simulink model "EX2_Pend_up_Controller_Observer"  (R2023b)
settings: Solver=FixedStepDiscrete  StartTime=0.0  StopTime=Inf  FixedStep=Ts  RelTol=1e-3  EnableMultiTasking=on
model workspace (MATLAB code in the model file):
  | % Processor Frequency
  | CPU_frequency = 90e6; %(Hz)
  | 
  | % PWM Settings
  | PWM_frequency = 15e3; %(Hz)
  | PWM_CounterPeriod = CPU_frequency/PWM_frequency/2; %(PWM timer counts)
  | 
  | % Switching frequency
  | fsw = PWM_frequency;
  | 
  | % Integration time (solver)
  | Ts = 1e-4;
  | 
  | % Encoder settings
  | fw = 400; % encoder sampling frequency
  | Tw = 1/fw; % encoder sampling time
values from neighbouring files (symbols this model uses):
  A = [0, 1, 0, 0 ... (first row only)    [EX2_init.m]
  Ad = sys_obs_disc.A    [EX2_init.m]
  B = Kf_avg * B    [EX2_init.m]
  Bd = sys_obs_disc.B    [EX2_init.m]
  C = [1, 0, 0, 0 ... (first row only)    [EX2_init.m]
  c_gains = K    [EX2_init.m]
  CALIBRATION_TIME = 50    [EX2_init.m]
  Cd = sys_obs_disc.C    [EX2_init.m]
  Dd = sys_obs_disc.D    [EX2_init.m]
  K = place(A, B, P_K)    [EX2_init.m]
  K_e = Distance / Encoder_Counts    (= 0.000124665903016)    [EX2_init.m]
  Lc = place(A', C', P_L)'    [EX2_init.m]
  SMC_switch = 1    [EX2_init.m]
  sys_params = [params.M, params.m, params.L, params.I, params.b_dynamic, params.bp_dynamic, params.g, K_sw]    [EX2_init.m]
undefined symbols (not defined in the file or in its folder): DiscIntNeverNeededParam, Down, GPTRIP1SEL, GPTRIP2SEL, TZ1, TZ2, Up
libraries: c2802xlib x5, eeGeneralControl x2, c2806xlib x2, dspstat3 x2, c280xlib x1, simulink x1, dspfdesign x1, dspsigops x1
settings Model: ExtModeTrigDuration=8  Creator=The MathWorks, Inc.  LastModifiedBy=98912
settings SolverCC: AlgebraicLoopSolver=TrustRegion  AutoInsertRateTranBlk=on
settings OptimizationCC: DefaultUnderspecifiedDataType=single  EnhancedBackFolding=on  PassReuseOutputArgsAs=Individual arguments  MaxStackSize=1024  OptimizeBlockOrder=speed  DifferentSizesBufferReuse=on  OptimizationCustomize=off  DenormalBehavior=FlushToZero  EfficientTunableParamExpr=on
settings DebuggingCC: ParameterTunabilityLossMsg=error  UnconnectedInputMsg=warning  UnconnectedOutputMsg=warning  UnconnectedLineMsg=warning  SubsystemReferenceDiagnosticForUnitTest=warning
settings HardwareCC: ProdBitPerChar=16  ProdBitPerInt=16  ProdBitPerPointer=32  ProdBitPerSizeT=32  ProdBitPerPtrDiffT=32  ProdLargestAtomicInteger=Integer  ProdLargestAtomicFloat=None  ProdWordSize=16  ProdLongLongMode=on  ProdHWDeviceType=Texas Instruments->C2000
settings ModelReferenceCC: EnableRefExpFcnMdlSchedulingChecks=on
settings SFSimCC: MATLABDynamicMemAlloc=off
settings RTWCC: Description=Embedded Coder  SystemTargetFile=ert.tlc  HardwareBoard=TI Piccolo F28069M LaunchPad  TemplateMakefile=ert_default_tmf  GenerateReport=on  Toolchain=Texas Instruments Code Composer Studio (C2000)  DLArmComputeVersion=19.05
settings CodeAppCC: ForceParamTrailComments=on  IgnoreCustomStorageClasses=off  OperatorAnnotations=on  SimulinkDataObjDesc=on  SFDataObjDesc=on  InsertBlockDesc=on
settings ERTTargetCC: CodeReplacementLibrary=TI C28x  ExtModeStaticAllocSize=2000
settings SettingsController: UseSoCProfilerForTargets=0

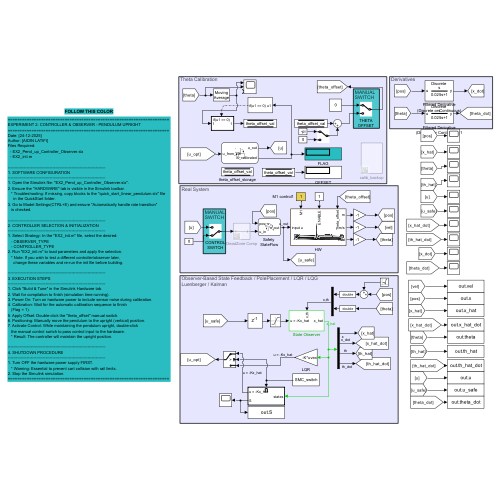
[thumbnail: Simulink's stored preview of the top-level diagram]
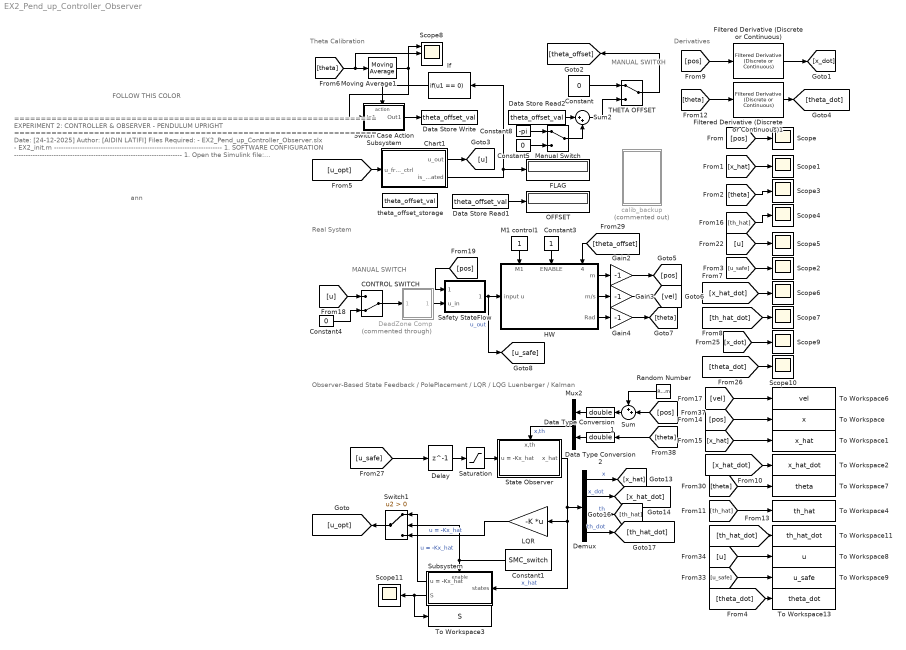
== system EX2_Pend_up_Controller_Observer ==
  note: FOLLOW THIS COLOR
  note: MANUAL
      | SWITCH
  note: MANUAL
      | SWITCH
  note: ====================================================================
      | EXPERIMENT 2: CONTROLLER & OBSERVER - PENDULUM UPRIGHT
      | ====================================================================
      | Date: [24-12-2025]
      | Author: [AIDIN LATIFI]
      | Files Required:
      |   - EX2_Pend_up_Controller_Observer.slx
      |   - EX2_init.m
      |
      | ------------------------------------------------------------------------
      | 1. SOFTWARE CONFIGURATION
      | ------------------------------------------------------------------------
      | 1. Open the Simulink file: "EX2_Pend_up_Controller_Observer.slx".
      | 2. Ensure the "HARDWARE" tab is visible in the Simulink toolbar.
      |    * Troubleshooting: If missing, copy blocks to the "quick_start_linear_pendulum.slx" file
      |      in the QuickStart folder.
      | 3. Go to Model Settings(CTRL+E) and ensure "Automatically handle rate transition"
      |    is checked.
      |
      | ------------------------------------------------------------------------
      | 2. CONTROLLER SELECTION & INITIALIZATION
      | ------------------------------------------------------------------------
      | 1. Select Strategy: In the "EX2_init.m" file, select the desired:
      |    - OBSERVER_TYPE
      |    - CONTROLLER_TYPE
      | 2. Run "EX2_init.m" to load parameters and apply the selection.
      |    * Note: If you wish to test a different controller/observer later,
      |      change these variables and re-run the init file before building.
      |
      | ------------------------------------------------------------------------
      | 3. EXECUTION STEPS
      | ------------------------------------------------------------------------
      | 1. Click "Build & Tune" in the Simulink Hardware tab.
      | 2. Wait for compilation to finish (simulation time running).
      | 3. Power On: Turn on hardware power to include sensor noise during calibration.
      | 4. Calibration: Wait for the automatic calibration sequence to finish
      |    (Flag = 1).
      | 5. Apply Offset: Double-click the "theta_offset" manual switch.
      | 6. Positioning: Manually move the pendulum to the upright (vertical) position.
      | 7. Activate Control: While maintaining the pendulum upright, double-click
      |    the manual control switch to pass control input to the hardware.
      |    * Result: The controller will maintain the upright position.
      |
      | ------------------------------------------------------------------------
      | 4. SHUTDOWN PROCEDURE
      | ------------------------------------------------------------------------
      | 1. Turn OFF the hardware power supply FIRST.
      |    * Warning: Essential to prevent cart collision with rail limits.
      | 2. Stop the Simulink simulation.
      | ====================================================================
  note: ann
  note: Theta Calibration
  note: Observer-Based State Feedback / PolePlacement / LQR / LQG
      | Luenberger / Kalman
  note: Real System
  note: Derivatives
  CONTROL SWITCH : ManualSwitch  CurrentSetting=0
  Chart1 : Stateflow chart  TreatAsAtomicUnit=on
  Constant : Constant  Value=0  SampleTime=Ts
  Constant1 : Constant  Value=SMC_switch
  Constant3 : Constant
  Constant4 : Constant  Value=0  SampleTime=-1
  Constant5 : Constant  Value=0  SampleTime=Ts
  Constant8 : Constant  Value=-pi  SampleTime=Ts
  Data Store Read1 : DataStoreRead  DataStoreName=theta_offset_val  IndexOptions=Index vector (dialog)  Indices=1  OutputSizes=1
  Data Store Read2 : DataStoreRead  DataStoreName=theta_offset_val  IndexOptions=Index vector (dialog)  Indices=1  OutputSizes=1
  Data Store Write : DataStoreWrite  DataStoreName=theta_offset_val  IndexOptions=Index vector (dialog)  Indices=1  OutputSizes=1
  Data Type Conversion1 : DataTypeConversion  OutDataTypeStr=double  SaturateOnIntegerOverflow=off  RndMeth=Floor
  Data Type Conversion2 : DataTypeConversion  OutDataTypeStr=double  SaturateOnIntegerOverflow=off  RndMeth=Floor
  DeadZone Comp : Subsystem  Commented=through
  Delay : Delay  DelayLength=1  SampleTime=Ts
  Demux : Demux
  FLAG : Display
  Filtered Derivative (Discrete or Continuous) : eeGeneralControl/Filtered Derivative (Discrete or Continuous)  K=1  T=0.025  B=inf  A=-inf  minRatio=10  init_option=Inherited from block input  x0=0  Ts=-1
      settings: LibrarySourceBlock=|
      | ee_sl_lib/General Control/Filtered Derivative
      | (Discrete or Continuous)
  Filtered Derivative (Discrete or Continuous)1 : eeGeneralControl/Filtered Derivative (Discrete or Continuous)  K=1  T=0.025  B=inf  A=-inf  minRatio=10  init_option=Inherited from block input  x0=0  Ts=-1
      settings: LibrarySourceBlock=|
      | ee_sl_lib/General Control/Filtered Derivative
      | (Discrete or Continuous)
  Gain2 : Gain  Gain=-1
  Gain3 : Gain  Gain=-1
  Gain4 : Gain  Gain=-1
  HW : Subsystem
      settings: PortSchema="{\"entries\":[{\"content\":{\"sides\":[{\"content\":{\"connectorIds\":[\"In1\"]},\"type\":\"ConnectorPlacement.EquallySpacedRectSide\",\"uuid\":\"e9898c75-a6e7-4646-b73a-b35b1fbe5adf\"},{\"content\":{\"connectorIds\":[\"Out1\",\"Out2\",\"Out3\"],\"side\":\"RIGHT\"},\"type\":\"ConnectorPlacement.EquallySpacedRectSide\",\"uuid\":\"085d2ccc-0e1f-4b16-8ec9-c70e62f660a1\"},{\"content\":{\"connectorIds\":[\"In2\",\"In3\",\"In4\"],\"side\":\"TOP\"},\"type\":\"ConnectorPlacement.EquallySpacedRectSide\",\"uuid\":\"51882789-74c2-4a7a-a001-ddaf25b9b479\"}]},\"type\":\"ConnectorPlacement.EquallySpacedConnector\",\"uuid\":\"373898fa-4a42-48b4-8ce1-77edd11dc4d5\"}],\"packageUris\":[\"http://schema.mathworks.com/mf0/Connector/R2020b\"],\"version\":\"1.0\"}"
      mask Display: image('lineer_pendulum_v2.jpg');
  If : If  IfExpression=u1 == 0  ShowElse=off
  LQR : Gain  Gain=-K  Multiplication=Matrix(K*u) (u vector)
  M1 control1 : Constant
  Manual Switch : ManualSwitch
  Moving Average1 : dspstat3/Moving Average  Method=Sliding window  ForgettingFactorPort=off  SpecifyWindowLength=off  WindowLength=200  OverlapLength=5  AllowArbitraryInputLength=off  ForgettingFactor=0.9  SimulateUsing=Interpreted execution
  Mux2 : Mux  Inputs=2
  OFFSET : Display
  Random Number : RandomNumber  Variance=1e-9
  Safety StateFlow : Stateflow chart  TreatAsAtomicUnit=on
  Saturation : Saturate  UpperLimit=1  LowerLimit=-1
  Scope{,1..7,9..11} (11 alike) : Scope
  Scope8 : Scope  NumInputPorts=3
  State Observer : Subsystem
      settings: PortSchema="{\"entries\":[{\"content\":{\"sides\":[{\"content\":{\"connectorIds\":[\"In1\"]},\"type\":\"ConnectorPlacement.EquallySpacedRectSide\",\"uuid\":\"78a5d6cc-05c3-4998-83bd-765592313900\"},{\"content\":{\"connectorIds\":[\"Out1\"],\"side\":\"RIGHT\"},\"type\":\"ConnectorPlacement.EquallySpacedRectSide\",\"uuid\":\"01493a4c-d438-46a2-bc76-28dd63b6a3eb\"},{\"content\":{\"connectorIds\":[\"In2\"],\"side\":\"TOP\"},\"type\":\"ConnectorPlacement.EquallySpacedRectSide\",\"uuid\":\"8eaa5f99-6d7d-4ceb-8f85-a6d0adbc0832\"}]},\"type\":\"ConnectorPlacement.EquallySpacedConnector\",\"uuid\":\"d4438f88-f341-4cd2-b661-553fe6a2df92\"}],\"packageUris\":[\"http://schema.mathworks.com/mf0/Connector/R2020b\"],\"version\":\"1.0\"}"
  Subsystem : Subsystem
  Sum : Sum  Inputs=++|
  Sum2 : Sum  Inputs=|++
  Switch Case Action Subsystem : Subsystem  TreatAsAtomicUnit=on
  Switch1 : Switch  Criteria=u2 > Threshold  SaturateOnIntegerOverflow=off  InputSameDT=off
  THETA OFFSET : ManualSwitch
  To Workspace : ToWorkspace  VariableName=x  SaveFormat=Timeseries  SampleTime=-1
  To Workspace1 : ToWorkspace  VariableName=x_hat  SaveFormat=Timeseries  SampleTime=-1
  To Workspace11 : ToWorkspace  VariableName=th_hat_dot  SaveFormat=Timeseries  SampleTime=-1
  To Workspace13 : ToWorkspace  VariableName=theta_dot  SaveFormat=Timeseries  SampleTime=-1
  To Workspace2 : ToWorkspace  VariableName=x_hat_dot  SaveFormat=Timeseries  SampleTime=-1
  To Workspace3 : ToWorkspace  VariableName=S  SaveFormat=Timeseries  SampleTime=-1
  To Workspace4 : ToWorkspace  VariableName=th_hat  SaveFormat=Timeseries  SampleTime=-1
  To Workspace6 : ToWorkspace  VariableName=vel  SaveFormat=Timeseries  SampleTime=-1
  To Workspace7 : ToWorkspace  VariableName=theta  SaveFormat=Timeseries  SampleTime=-1
  To Workspace8 : ToWorkspace  VariableName=u  SaveFormat=Timeseries  SampleTime=-1
  To Workspace9 : ToWorkspace  VariableName=u_safe  SaveFormat=Timeseries  SampleTime=-1
  calib_backup : Subsystem  Commented=on
  theta_offset_storage : DataStoreMemory  DataStoreName=theta_offset_val  WriteAfterWriteMsg=warning  ShowAdditionalParam=off
  wires:
  [u_safe] -> Scope2/1
  Constant8/1 -> Manual Switch/1
  If/1 -> Switch Case Action Subsystem/Action
  [u_opt] -> Chart1/1(u_from_ctrl)
  [theta] -> Filtered Derivative (Discrete or Continuous)1/1
  Constant/1 -> THETA OFFSET/1
  Constant4/1 -> CONTROL SWITCH/2
  THETA OFFSET/1 -> [theta_offset]
  Sum2/1 -> THETA OFFSET/2
  [th_hat_dot] -> To Workspace11/1
  [theta] -> Scope8/2, Moving Average1/1
  [theta] -> Data Type Conversion2/1
  Switch Case Action Subsystem/1(Out1) -> Data Store Write/1
  [x_hat_dot] -> To Workspace2/1
  Manual Switch/1 -> Sum2/2
  Safety StateFlow/1(u_out) -> HW/1(input u), [u_safe]  "u_out"
  HW/3(Rad) -> Gain4/1
  Chart1/2(is_calibrated) -> FLAG/1, If/1
  [th_hat] -> To Workspace4/1
  Sum/1 -> Data Type Conversion1/1
  [pos] -> To Workspace/1
  Constant3/1 -> HW/3(ENABLE)
  M1 control1/1 -> HW/2(M1)
  Random Number/1 -> Sum/1
  Demux/1 -> [x_hat]  "x"
  [u] -> Scope5/1
  [x_hat] -> To Workspace1/1
  Demux/2 -> [x_hat_dot]  "x_dot"
  CONTROL SWITCH/1 -> DeadZone Comp/1(In1)
  [pos] -> Scope/1
  HW/2(m/s) -> Gain3/1
  [pos] -> Sum/2
  LQR/1 -> Switch1/3  "u = -Kx_hat"
  Gain3/1 -> [vel]
  Chart1/1(u_out) -> [u]
  Filtered Derivative (Discrete or Continuous)/1 -> [x_dot]
  Gain2/1 -> [pos]
  [th_hat_dot] -> Scope7/1
  Constant5/1 -> Manual Switch/2
  [pos] -> Filtered Derivative (Discrete or Continuous)/1
  [theta_offset] -> HW/4(Theta_offset)
  Moving Average1/1 -> Switch Case Action Subsystem/1(In1), Scope8/1
  Filtered Derivative (Discrete or Continuous)1/1 -> [theta_dot]
  Gain4/1 -> [theta]
  Data Store Read1/1 -> OFFSET/1
  [u_safe] -> To Workspace9/1
  [theta] -> Scope3/1
  [x_hat_dot] -> Scope6/1
  [pos] -> Safety StateFlow/1(pos_s)
  [x_hat] -> Scope1/1
  State Observer/1(x_hat) -> LQR/1, Subsystem/1(states), Demux/1  "x_hat"
  Demux/4 -> [th_hat_dot]  "th_dot"
  [th_hat] -> Scope4/1
  Data Type Conversion2/1 -> Mux2/2
  Mux2/1 -> State Observer/2(x,th)  "x,th"
  [vel] -> To Workspace6/1
  HW/1(m) -> Gain2/1
  [u] -> CONTROL SWITCH/1
  DeadZone Comp/1(Out1) -> Safety StateFlow/2(u_in)
  [x_dot] -> Scope9/1
  Data Type Conversion1/1 -> Mux2/1
  [theta_dot] -> To Workspace13/1
  [theta_dot] -> Scope10/1
  [theta] -> To Workspace7/1
  Demux/3 -> [th_hat]  "th"
  [u] -> To Workspace8/1
  Data Store Read2/1 -> Sum2/1
  Delay/1 -> Saturation/1
  [u_safe] -> Delay/1
  Saturation/1 -> State Observer/1(u = -Kx_hat)
  Constant1/1 -> Subsystem/Enable, Switch1/2
  Subsystem/2(S) -> To Workspace3/1, Scope11/1
  Subsystem/1(u = -Kx_hat) -> Switch1/1  "u = -Kx_hat"
  Switch1/1 -> [u_opt]

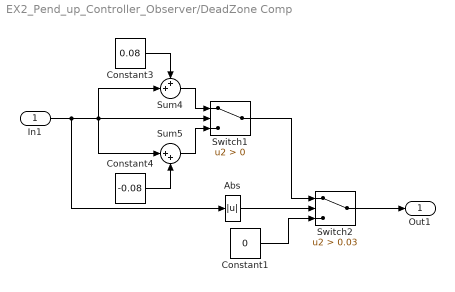
== system EX2_Pend_up_Controller_Observer/DeadZone Comp ==
  In1 : Inport
  Abs : Abs  SaturateOnIntegerOverflow=off
  Constant1 : Constant  Value=0  SampleTime=Ts
  Constant3 : Constant  Value=0.08  SampleTime=Ts
  Constant4 : Constant  Value=-0.08  SampleTime=Ts
  Sum4 : Sum  Inputs=++|
  Sum5 : Sum  Inputs=|++
  Switch1 : Switch  Criteria=u2 > Threshold  ZeroCross=off  SaturateOnIntegerOverflow=off  InputSameDT=off
  Switch2 : Switch  Criteria=u2 > Threshold  Threshold=0.03  ZeroCross=off  SaturateOnIntegerOverflow=off  InputSameDT=off
  Out1 : Outport
  wires:
  Switch2/1 -> Out1/1
  Constant1/1 -> Switch2/3
  Abs/1 -> Switch2/2
  In1/1 -> Abs/1, Switch1/2, Sum4/2, Sum5/1
  Constant4/1 -> Sum5/2
  Sum4/1 -> Switch1/1
  Switch1/1 -> Switch2/1
  Sum5/1 -> Switch1/3
  Constant3/1 -> Sum4/1

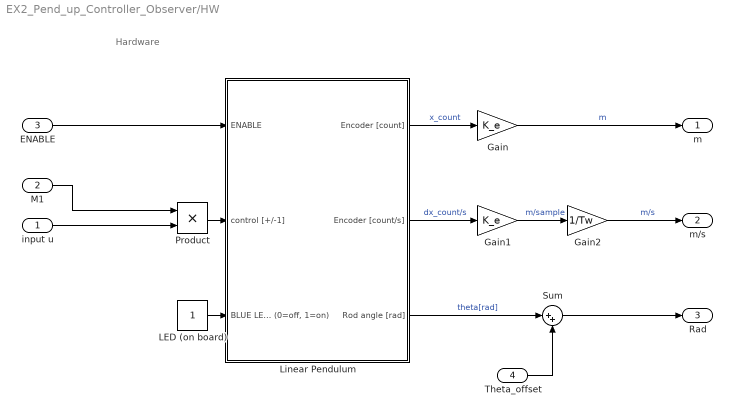
== system EX2_Pend_up_Controller_Observer/HW ==
  note: Hardware
  input u : Inport
  M1 : Inport  Port=2
  ENABLE : Inport  Port=3
  Theta_offset : Inport  Port=4
  Gain : Gain  Gain=K_e
  Gain1 : Gain  Gain=K_e
  Gain2 : Gain  Gain=1/Tw
  LED (on board) : Constant  SampleTime=0.5
  Linear Pendulum : Subsystem
  Product : Product
  Sum : Sum  Inputs=|++
  m : Outport
  m/s : Outport  Port=2
  Rad : Outport  Port=3
  wires:
  Sum/1 -> Rad/1
  Gain1/1 -> Gain2/1  "m/sample"
  Theta_offset/1 -> Sum/2
  Gain/1 -> m/1  "m"
  Gain2/1 -> m/s/1  "m/s"
  M1/1 -> Product/1
  Linear Pendulum/2(Encoder [count/s]) -> Gain1/1  "dx_count/s"
  input u/1 -> Product/2
  Linear Pendulum/3(Rod angle [rad]) -> Sum/1  "theta[rad]"
  Product/1 -> Linear Pendulum/2(control [+/-1])
  LED (on board)/1 -> Linear Pendulum/3("BLUE LED (0=off, 1=on)")
  Linear Pendulum/1(Encoder [count]) -> Gain/1  "x_count"
  ENABLE/1 -> Linear Pendulum/1(ENABLE)

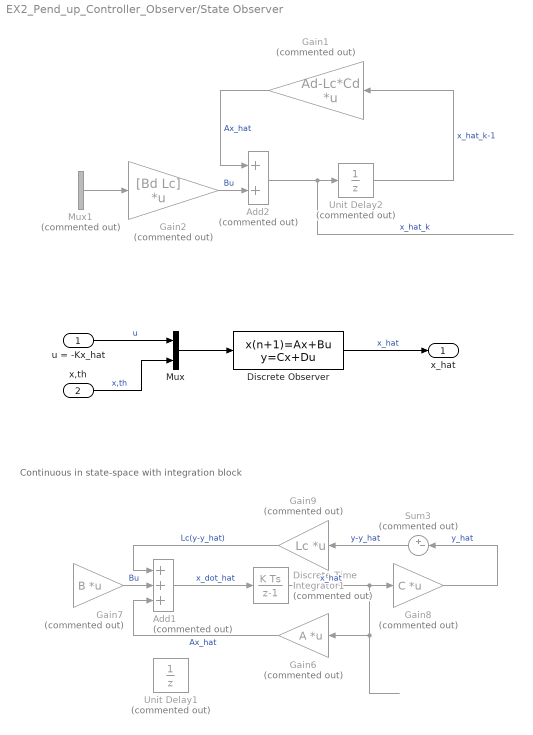
== system EX2_Pend_up_Controller_Observer/State Observer ==
  note: Continuous in state-space with integration block
  u = -Kx_hat : Inport
  x,th : Inport  Port=2
  Add1 : Sum  Commented=on  Inputs=+++
  Add2 : Sum  Commented=on
  Discrete Observer : DiscreteStateSpace  A=Ad  B=Bd  C=Cd  D=Dd  InitialCondition=[0;0;0;0]  SampleTime=Ts
  Discrete-Time Integrator1 : DiscreteIntegrator  Commented=on  InitialCondition=[0,0,0,0]  SampleTime=-1  LimitOutput=on  UpperSaturationLimit=0.01  LowerSaturationLimit=-0.01  ICPrevOutput=DiscIntNeverNeededParam  ICPrevScaledInput=DiscIntNeverNeededParam
  Gain1 : Gain  Commented=on  Gain=Ad-Lc*Cd  Multiplication=Matrix(K*u) (u vector)
  Gain2 : Gain  Commented=on  Gain=[Bd Lc]  Multiplication=Matrix(K*u) (u vector)
  Gain6 : Gain  Commented=on  Gain=A  Multiplication=Matrix(K*u) (u vector)
  Gain7 : Gain  Commented=on  Gain=B  Multiplication=Matrix(K*u) (u vector)
  Gain8 : Gain  Commented=on  Gain=C  Multiplication=Matrix(K*u) (u vector)
  Gain9 : Gain  Commented=on  Gain=Lc  Multiplication=Matrix(K*u) (u vector)
  Mux : Mux  Inputs=2
  Mux1 : Mux  Commented=on  Inputs=2
  Sum3 : Sum  Commented=on  Inputs=+-|
  Unit Delay1 : UnitDelay  Commented=on  SampleTime=-1  HasFrameUpgradeWarning=on
  Unit Delay2 : UnitDelay  Commented=on  SampleTime=-1  HasFrameUpgradeWarning=on
  x_hat : Outport
  wires:
  Gain6/1 -> Add1/3  "Ax_hat"
  Sum3/1 -> Gain9/1  "y-y_hat"
  Gain8/1 -> Sum3/2  "y_hat"
  Gain9/1 -> Add1/1  "Lc(y-y_hat)"
  Gain7/1 -> Add1/2  "Bu"
  Add1/1 -> Discrete-Time Integrator1/1  "x_dot_hat"
  Discrete-Time Integrator1/1 -> Gain6/1, Gain8/1  "x_hat"
  Mux/1 -> Discrete Observer/1
  Discrete Observer/1 -> x_hat/1  "x_hat"
  x,th/1 -> Mux/2  "x,th"
  u = -Kx_hat/1 -> Mux/1  "u"
  ? -> Sum3/1  "x,th"
  ? -> Gain7/1  "u"
  Add2/1 -> Unit Delay2/1  "x_hat_k"
  Gain2/1 -> Add2/2  "Bu"
  Gain1/1 -> Add2/1  "Ax_hat"
  Mux1/1 -> Gain2/1
  Unit Delay2/1 -> Gain1/1  "x_hat_k-1"
  ? -> Mux1/2  "x,th"
  ? -> Mux1/1  "u"

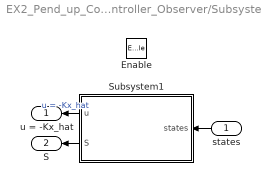
== system EX2_Pend_up_Controller_Observer/Subsystem ==
  states : Inport
  Enable : EnablePort
  Subsystem1 : Subsystem  mask{sys_params=sys_params, c_gains=c_gains}
      mask prompts: sys_params "(M, m, l, g): sys params"; c_gains "(c1, c2, c3, c4): C gains"
      mask DialogControl DescTextVar Prompt: Input parameters for custom SMC
  u = -Kx_hat : Outport
  S : Outport  Port=2
  wires:
  states/1 -> Subsystem1/1(states)
  Subsystem1/2(S) -> S/1
  Subsystem1/1(u) -> u = -Kx_hat/1  "u = -Kx_hat"

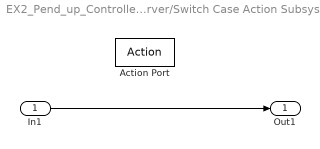
== system EX2_Pend_up_Controller_Observer/Switch Case Action Subsystem ==
  In1 : Inport
  Action Port : ActionPort  ActionPortLabel=if(u1 == 0)
  Out1 : Outport
  wires:
  In1/1 -> Out1/1

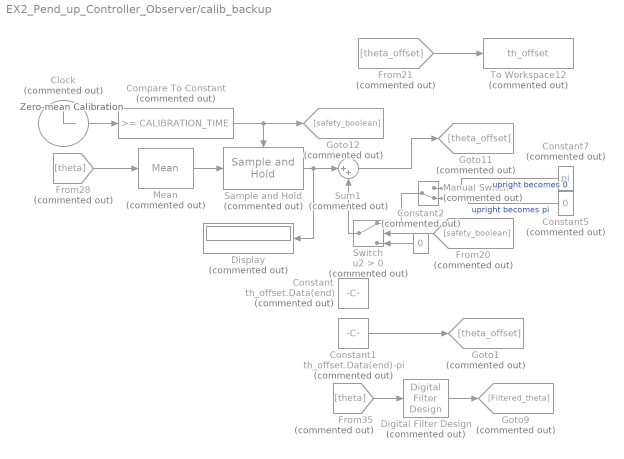
== system EX2_Pend_up_Controller_Observer/calib_backup ==
  note: Zero-mean Calibration
  Clock : Clock  Commented=on
  Compare To Constant : simulink/Logic and Bit Operations/Compare To Constant  Commented=on  relop=>=  const=CALIBRATION_TIME  OutDataTypeStr=boolean
  Constant : Constant  Commented=on  Value=th_offset.Data(end)
  Constant1 : Constant  Commented=on  Value=th_offset.Data(end)-pi
  Constant2 : Constant  Commented=on  Value=0  SampleTime=-1
  Constant5 : Constant  Commented=on  Value=0  SampleTime=-1
  Constant7 : Constant  Commented=on  Value=pi  SampleTime=-1
  Digital Filter Design : dspfdesign/Digital Filter Design  Commented=on  mwdsp_browser_bugfix_var=off
  Display : Display  Commented=on
  From20 : From  Commented=on  GotoTag=safety_boolean
  From21 : From  Commented=on  GotoTag=theta_offset
  From28 : From  Commented=on  GotoTag=theta
  From35 : From  Commented=on  GotoTag=theta
  Goto1 : Goto  Commented=on  GotoTag=theta_offset
  Goto11 : Goto  Commented=on  GotoTag=theta_offset
  Goto12 : Goto  Commented=on  GotoTag=safety_boolean
  Goto9 : Goto  Commented=on  GotoTag=Filtered_theta
  Manual Switch4 : ManualSwitch  Commented=on  CurrentSetting=0
  Mean : dspstat3/Mean  Commented=on  run=off  InputProcessing=Columns as channels (frame based)  reset_popup=None  directionMode=Each column  dimension=1  roiEnable=off  roiType=Rectangles  roiPortion=Entire ROI  roiOutput=Individual statistics for each ROI  roiFlag=off  roundingMode=Floor  overflowMode=off  outputDataTypeStr=Inherit: Same as accumulator  outputMin=[]  outputMax=[]  outputLastDataTypeStr=Inherit: Same as accumulator
  Sample and Hold : dspsigops/Sample and Hold  Commented=on  trig=Rising edge  initCond=0  latchinput=on
  Sum1 : Sum  Commented=on  Inputs=|++
  Switch : Switch  Commented=on  Criteria=u2 > Threshold  SaturateOnIntegerOverflow=off  InputSameDT=off
  To Workspace12 : ToWorkspace  Commented=on  VariableName=th_offset  SaveFormat=Timeseries  SampleTime=-1
  wires:
  Constant1/1 -> Goto1/1
  Compare To Constant/1 -> Sample and Hold/Trigger, Goto12/1
  Digital Filter Design/1 -> Goto9/1
  Sum1/1 -> Goto11/1
  Sample and Hold/1 -> Display/1, Sum1/1
  From28/1 -> Mean/1
  Switch/1 -> Sum1/2
  Mean/1 -> Sample and Hold/1
  From35/1 -> Digital Filter Design/1
  From21/1 -> To Workspace12/1
  Constant2/1 -> Switch/3
  Constant7/1 -> Manual Switch4/1  "upright becomes 0"
  Clock/1 -> Compare To Constant/1
  Constant5/1 -> Manual Switch4/2  "upright becomes pi"
  From20/1 -> Switch/2
  Manual Switch4/1 -> Switch/1

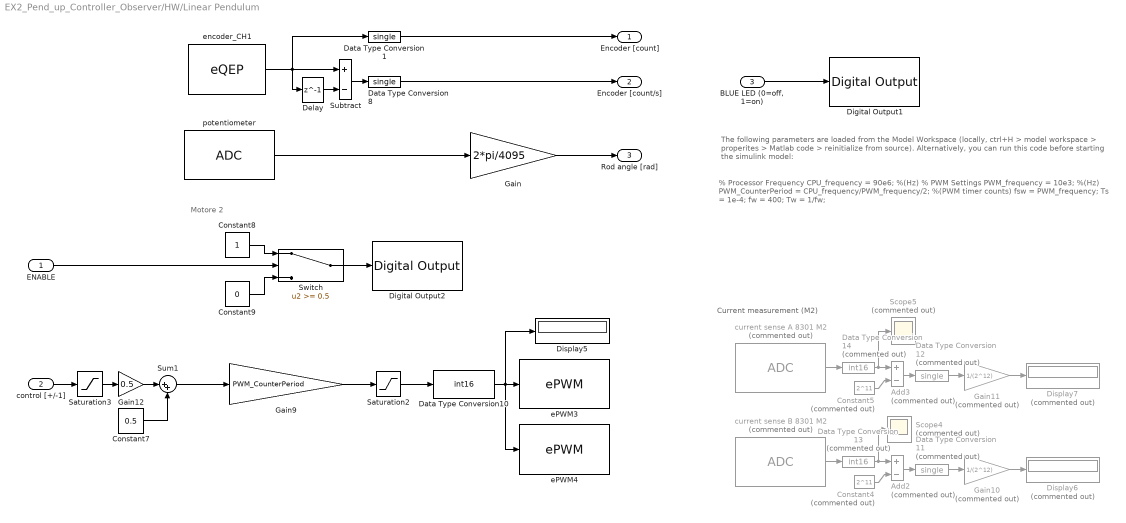
== system EX2_Pend_up_Controller_Observer/HW/Linear Pendulum ==
  note: Current measurement (M2)
  note: The following parameters are loaded from the Model Workspace (locally, ctrl+H > model workspace > properites > Matlab code > reinitialize from source). Alternatively, you can run this code before starting the simulink model:
  note: % Processor Frequency
      | CPU_frequency = 90e6; %(Hz)
      | % PWM Settings
      | PWM_frequency = 10e3; %(Hz)
      | PWM_CounterPeriod = CPU_frequency/PWM_frequency/2; %(PWM timer counts)
      | fsw = PWM_frequency;
      | Ts = 1e-4;
      | fw = 400;
      | Tw = 1/fw;
  note: Motore 2
  ENABLE : Inport
  control [+/-1] : Inport  Port=2
  "BLUE LED (0=off, 1=on)" : Inport  Port=3
  Add2 : Sum  Commented=on  Inputs=+-
  Add3 : Sum  Commented=on  Inputs=+-
  Constant4 : Constant  Commented=on  Value=2^11  OutDataTypeStr=int16  SampleTime=Ts*10
  Constant5 : Constant  Commented=on  Value=2^11  OutDataTypeStr=int16  SampleTime=Ts*10
  Constant7 : Constant  Value=0.5
  Constant8 : Constant
  Constant9 : Constant  Value=0
  Data Type Conversion1 : DataTypeConversion  OutDataTypeStr=single  SaturateOnIntegerOverflow=off  RndMeth=Floor
  Data Type Conversion10 : DataTypeConversion  OutDataTypeStr=int16  SaturateOnIntegerOverflow=off  RndMeth=Floor
  Data Type Conversion11 : DataTypeConversion  Commented=on  OutDataTypeStr=single  SaturateOnIntegerOverflow=off  RndMeth=Floor
  Data Type Conversion12 : DataTypeConversion  Commented=on  OutDataTypeStr=single  SaturateOnIntegerOverflow=off  RndMeth=Floor
  Data Type Conversion13 : DataTypeConversion  Commented=on  OutDataTypeStr=int16  SaturateOnIntegerOverflow=off  RndMeth=Floor
  Data Type Conversion14 : DataTypeConversion  Commented=on  OutDataTypeStr=int16  SaturateOnIntegerOverflow=off  RndMeth=Floor
  Data Type Conversion8 : DataTypeConversion  OutDataTypeStr=single  SaturateOnIntegerOverflow=off  RndMeth=Floor
  Delay : Delay  DelayLength=1  SampleTime=Tw
  Digital Output1 : c2806xlib/Digital Output  GPIO_Number=GPIO32~GPIO39  GPIO_Bit0=off  GPIO_BIT0_Toggle=off  GPIO_Bit1=off  GPIO_BIT1_Toggle=off  GPIO_Bit2=off  GPIO_BIT2_Toggle=off  GPIO_Bit3=off  GPIO_BIT3_Toggle=off  GPIO_Bit4=off  GPIO_BIT4_Toggle=off  GPIO_Bit5=off  GPIO_BIT5_Toggle=off  GPIO_Bit6=off  GPIO_BIT6_Toggle=off  GPIO_Bit7=on  GPIO_BIT7_Toggle=on
  Digital Output2 : c2806xlib/Digital Output  GPIO_Number=GPIO8~GPIO15  GPIO_Bit0=off  GPIO_BIT0_Toggle=off  GPIO_Bit1=off  GPIO_BIT1_Toggle=off  GPIO_Bit2=off  GPIO_BIT2_Toggle=off  GPIO_Bit3=off  GPIO_BIT3_Toggle=off  GPIO_Bit4=on  GPIO_BIT4_Toggle=off  GPIO_Bit5=off  GPIO_BIT5_Toggle=off  GPIO_Bit6=off  GPIO_BIT6_Toggle=off  GPIO_Bit7=off  GPIO_BIT7_Toggle=off
  Display5 : Display
  Display6 : Display  Commented=on
  Display7 : Display  Commented=on
  Gain : Gain  Gain=2*pi/4095
  Gain10 : Gain  Commented=on  Gain=1/(2^12)
  Gain11 : Gain  Commented=on  Gain=1/(2^12)
  Gain12 : Gain  Gain=0.5
  Gain9 : Gain  Gain=PWM_CounterPeriod
  Saturation2 : Saturate  UpperLimit=PWM_CounterPeriod  LowerLimit=0
  Saturation3 : Saturate  UpperLimit=1  LowerLimit=-1
  Scope4 : Scope  Commented=on
  Scope5 : Scope  Commented=on
  Subtract : Sum  Inputs=+-
  Sum1 : Sum  Inputs=|++
  Switch : Switch  Threshold=0.5  SaturateOnIntegerOverflow=off  InputSameDT=off
  current sense A 8301 M2 : c2802xlib/ADC  Commented=on  blkParamProc=C2000  ADCModule=1  samplingMode=Single sample mode  ADCResolution=12-bit (Single-ended input)  useSOC1=SOC3  useSOC2=SOC0_SOC1  SOCAcquisitionWindow=7  SOCTriggerSource=ePWM4_ADCSOCA  SOCInterruptTrigger=No ADCINT  Ts=Ts*10  dType=uint16  postInterrupt=off  interruptSel=ADCINT1  ADCINTContinuous=on  endma=off  chdma=1  conv1=ADCINA3  conv2=ADCINA0 and ADCINB0  conv1_Type4=ADCIN0  conv2_Type4=ADCIN0 and ADCIN1
  current sense B 8301 M2 : c2802xlib/ADC  Commented=on  blkParamProc=C2000  ADCModule=1  samplingMode=Single sample mode  ADCResolution=12-bit (Single-ended input)  useSOC1=SOC4  useSOC2=SOC0_SOC1  SOCAcquisitionWindow=7  SOCTriggerSource=ePWM5_ADCSOCA  SOCInterruptTrigger=No ADCINT  Ts=Ts*10  dType=uint16  postInterrupt=off  interruptSel=ADCINT1  ADCINTContinuous=on  endma=off  chdma=1  conv1=ADCINB3  conv2=ADCINA0 and ADCINB0  conv1_Type4=ADCIN0  conv2_Type4=ADCIN0 and ADCIN1
  ePWM3 : c2802xlib/ePWM  PwmType=C2000  useModule=ePWM1  ePWMxLINKTBPRD=Not Linked  periodUnits=Clock cycles  timerSource=Specify via dialog  timerPeriod_clk=PWM_CounterPeriod+1  timerPeriod_sec=0.0001  tbshadow=Counter equals to zero  countingMode=Up-Down  phaseActiveEnable=Disable  phaseDirection=Count down after sync  phaseActive=0  synchronizationEnable=off  dcaevt1Sync=off  dcbevt1Sync=off  synchronizationOption=Disable  dcbevt1SyncOut=off  dcaevt1SyncOut=off  cmpdSyncOut=off  cmpcSyncOut=off  cmpbSyncOut=off  zeroSyncOut=off  swfSyncOut=off  perSynchronizationOption=Counter equals to period (CTR=PRD)  clockPrescale=1  HSclockPrescale=1  enswap=off  ePWMxAStatus=on  ePWMxAactionLogic1=Do nothing  ePWMxAactionLogic2=Do nothing  ePWMxAactionLogic3=Clear  ePWMxAactionLogic4=Set  ePWMxAactionLogic5=Do nothing  ePWMxAactionLogic6=Do nothing  ePWMxACSFenable=off  ePWMxACSFvalue=Forcing disable  ePWMxASFreload=Zero  ePWMxBStatus=off  ePWMxBactionLogic1=Set  ePWMxBactionLogic2=Clear  ePWMxBactionLogic3=Do nothing  ePWMxBactionLogic4=Do nothing  ePWMxBactionLogic5=Clear  ePWMxBactionLogic6=Set  ePWMxBCSFenable=off  ePWMxBCSFvalue=Forcing disable  ePWMxBSFreload=Zero  ePWNxBOutWay=on  ePWMxLINKCMPA=Not Linked  CMPAUnits=Clock cycles  CMPASource=Input port  CMPAValue_per=50  CMPAValue_clk=PWM_CounterPeriod/2+1  enCMPAshadow=Counter equals to zero (CTR=Zero)  ePWMxLINKCMPB=Not Linked  CMPBUnits=Clock cycles  CMPBSource=Specify via dialog  CMPBValue_per=50  CMPBValue_clk=PWM_CounterPeriod/2 +1  enCMPBshadow=Counter equals to zero (CTR=Zero)  ePWMxLINKCMPC=Not Linked  CMPCUnits=Clock cycles  CMPCSource=Specify via dialog  CMPCValue_per=50  CMPCValue_clk=32000  enCMPCshadow=Counter equals to zero (CTR=Zero)  ePWMxLINKCMPD=Not Linked  CMPDUnits=Clock cycles  CMPDSource=Specify via dialog  CMPDValue_per=50  CMPDValue_clk=32000  enCMPDshadow=Counter equals to zero (CTR=Zero)  enableDBePWMxA=on  enableDBePWMxB=on  enhalfcycle=off  DBpolarity=Active high (AH)  DBedgeDelay=Positive  DBSource_ePWMxA=ePWMxA  DBSource_ePWMxB=ePWMxA  DBPeriodUnits=Clock cycles  DBperiodSource=Specify via dialog  REDperiod=15  FEDperiod=15  REDperiod_sec=0  FEDperiod_sec=0  LoadModeDBRED=Immediate without using shadow  LoadModeDBFED=Immediate without using shadow  adcstartModuleA=on  adcrequestEventA=First event  adcstartEventA=Counter equals to period (CTR=PRD)  adcstartEventA_type2=Digital Compare Module A Event 1 start of conversion (DCAEVT1.soc)  adcstartModuleB=off  adcrequestEventB=First event  adcstartEventB=Counter equals to zero (CTR=Zero)  adcstartEventB_type2=Counter equals to zero (CTR=Zero)  intEn=off  intPrd=First event  intSel=Counter equals to zero (CTR=Zero)  intSel_type2=Counter equals to zero (CTR=Zero)  hrpe=off  enHRPWM=off  HRPWM_LoadMode=Counter equals to period (CTR=PRD)  HRPWM_CTLMode=Duty or Period control mode  HRPWM_EDGMode=Both edge  hrpeb=off  enHRPWMB=off  HRPWM_LoadModeB=Counter equals to zero (CTR=ZERO)  HRPWM_CTLModeB=Duty or Period control mode  HRPWM_EDGModeB=Both edge  enHRDBRED=off  enHRDBFED=off  enSFO=on  enautoconv=on  chopperEnable=off  chopperFrequency=1  chopperFirstwidth=1  chopperDuty=12.5%  tripZonesource=Specify via dialog  tzselOSHT1=off  tzselOSHT2=off  tzselOSHT3=off  tzselOSHT4=off  tzselOSHT5=off  tzselOSHT6=off  tzselOSHDCAEV1=off  tzselOSHDCBEV1=off  tzselCBC1=off  tzselCBC2=off  tzselCBC3=off  tzselCBC4=off  tzselCBC5=off  tzselCBC6=off  tzselCBCDCAEV2=off  tzselCBCDCBEV2=off  enTzOstIntr=off  enTzCbcIntr=off  enTzDCAEVT1Intr=off  enTzDCAEVT2Intr=off  enTzDCBEVT1Intr=off  enTzDCBEVT2Intr=off  tzclrCBCLatch=Counter equals to zero (CTR=Zero)  ePWMxAforced=No action  ePWMxBforced=No action  DCAEVT1forced=No action  DCBEVT1forced=No action  DCAEVT2forced=No action  DCBEVT2forced=No action  dcah=Trip Zone 1 input (TZ1)  dcal=Trip Zone 2 input (TZ2)  dcbh=Trip Zone 1 input (TZ1)  dcbl=Trip Zone 2 input (TZ2)  dcah_type2=GPTRIP1SEL/(TZ1)  dcal_type2=GPTRIP2SEL/(TZ2)  dcbh_type2=GPTRIP1SEL/(TZ1)  dcbl_type2=GPTRIP2SEL/(TZ2)  gendcaevt1=Event disabled  gendcaevt2=Event disabled  gendcbevt1=Event disabled  gendcbevt2=Event disabled  dcaevt1src=DCAEVT1 with sync  dcaevt2src=DCAEVT2 with sync  dcbevt1src=DCBEVT1 with sync  dcbevt2src=DCBEVT2 with sync  pulsesel=Counter equals to zero (CTR=Zero)  blankinv=off  blankoffset=0  blankwidth=0  evsrcsel=Filtered version of DCAEVT1 (DCAEVT1FILT)  encape=off
  ePWM4 : c2802xlib/ePWM  PwmType=C2000  useModule=ePWM2  ePWMxLINKTBPRD=Not Linked  periodUnits=Clock cycles  timerSource=Specify via dialog  timerPeriod_clk=PWM_CounterPeriod+1  timerPeriod_sec=0.0001  tbshadow=Counter equals to zero  countingMode=Up-Down  phaseActiveEnable=Disable  phaseDirection=Count down after sync  phaseActive=0  synchronizationEnable=off  dcaevt1Sync=off  dcbevt1Sync=off  synchronizationOption=Disable  dcbevt1SyncOut=off  dcaevt1SyncOut=off  cmpdSyncOut=off  cmpcSyncOut=off  cmpbSyncOut=off  zeroSyncOut=off  swfSyncOut=off  perSynchronizationOption=Counter equals to period (CTR=PRD)  clockPrescale=1  HSclockPrescale=1  enswap=on  ePWMxAStatus=on  ePWMxAactionLogic1=Do nothing  ePWMxAactionLogic2=Do nothing  ePWMxAactionLogic3=Clear  ePWMxAactionLogic4=Set  ePWMxAactionLogic5=Do nothing  ePWMxAactionLogic6=Do nothing  ePWMxACSFenable=off  ePWMxACSFvalue=Forcing disable  ePWMxASFreload=Zero  ePWMxBStatus=off  ePWMxBactionLogic1=Set  ePWMxBactionLogic2=Clear  ePWMxBactionLogic3=Do nothing  ePWMxBactionLogic4=Do nothing  ePWMxBactionLogic5=Clear  ePWMxBactionLogic6=Set  ePWMxBCSFenable=off  ePWMxBCSFvalue=Forcing disable  ePWMxBSFreload=Zero  ePWNxBOutWay=on  ePWMxLINKCMPA=Not Linked  CMPAUnits=Clock cycles  CMPASource=Input port  CMPAValue_per=50  CMPAValue_clk=PWM_CounterPeriod/2+1  enCMPAshadow=Counter equals to zero (CTR=Zero)  ePWMxLINKCMPB=Not Linked  CMPBUnits=Clock cycles  CMPBSource=Specify via dialog  CMPBValue_per=50  CMPBValue_clk=PWM_CounterPeriod/2 +1  enCMPBshadow=Counter equals to zero (CTR=Zero)  ePWMxLINKCMPC=Not Linked  CMPCUnits=Clock cycles  CMPCSource=Specify via dialog  CMPCValue_per=50  CMPCValue_clk=32000  enCMPCshadow=Counter equals to zero (CTR=Zero)  ePWMxLINKCMPD=Not Linked  CMPDUnits=Clock cycles  CMPDSource=Specify via dialog  CMPDValue_per=50  CMPDValue_clk=32000  enCMPDshadow=Counter equals to zero (CTR=Zero)  enableDBePWMxA=on  enableDBePWMxB=on  enhalfcycle=off  DBpolarity=Active high (AH)  DBedgeDelay=Positive  DBSource_ePWMxA=ePWMxA  DBSource_ePWMxB=ePWMxA  DBPeriodUnits=Clock cycles  DBperiodSource=Specify via dialog  REDperiod=15  FEDperiod=15  REDperiod_sec=0  FEDperiod_sec=0  LoadModeDBRED=Immediate without using shadow  LoadModeDBFED=Immediate without using shadow  adcstartModuleA=on  adcrequestEventA=First event  adcstartEventA=Counter equals to period (CTR=PRD)  adcstartEventA_type2=Digital Compare Module A Event 1 start of conversion (DCAEVT1.soc)  adcstartModuleB=off  adcrequestEventB=First event  adcstartEventB=Counter equals to zero (CTR=Zero)  adcstartEventB_type2=Counter equals to zero (CTR=Zero)  intEn=off  intPrd=First event  intSel=Counter equals to zero (CTR=Zero)  intSel_type2=Counter equals to zero (CTR=Zero)  hrpe=off  enHRPWM=off  HRPWM_LoadMode=Counter equals to period (CTR=PRD)  HRPWM_CTLMode=Duty or Period control mode  HRPWM_EDGMode=Both edge  hrpeb=off  enHRPWMB=off  HRPWM_LoadModeB=Counter equals to zero (CTR=ZERO)  HRPWM_CTLModeB=Duty or Period control mode  HRPWM_EDGModeB=Both edge  enHRDBRED=off  enHRDBFED=off  enSFO=on  enautoconv=on  chopperEnable=off  chopperFrequency=1  chopperFirstwidth=1  chopperDuty=12.5%  tripZonesource=Specify via dialog  tzselOSHT1=off  tzselOSHT2=off  tzselOSHT3=off  tzselOSHT4=off  tzselOSHT5=off  tzselOSHT6=off  tzselOSHDCAEV1=off  tzselOSHDCBEV1=off  tzselCBC1=off  tzselCBC2=off  tzselCBC3=off  tzselCBC4=off  tzselCBC5=off  tzselCBC6=off  tzselCBCDCAEV2=off  tzselCBCDCBEV2=off  enTzOstIntr=off  enTzCbcIntr=off  enTzDCAEVT1Intr=off  enTzDCAEVT2Intr=off  enTzDCBEVT1Intr=off  enTzDCBEVT2Intr=off  tzclrCBCLatch=Counter equals to zero (CTR=Zero)  ePWMxAforced=No action  ePWMxBforced=No action  DCAEVT1forced=No action  DCBEVT1forced=No action  DCAEVT2forced=No action  DCBEVT2forced=No action  dcah=Trip Zone 1 input (TZ1)  dcal=Trip Zone 2 input (TZ2)  dcbh=Trip Zone 1 input (TZ1)  dcbl=Trip Zone 2 input (TZ2)  dcah_type2=GPTRIP1SEL/(TZ1)  dcal_type2=GPTRIP2SEL/(TZ2)  dcbh_type2=GPTRIP1SEL/(TZ1)  dcbl_type2=GPTRIP2SEL/(TZ2)  gendcaevt1=Event disabled  gendcaevt2=Event disabled  gendcbevt1=Event disabled  gendcbevt2=Event disabled  dcaevt1src=DCAEVT1 with sync  dcaevt2src=DCAEVT2 with sync  dcbevt1src=DCBEVT1 with sync  dcbevt2src=DCBEVT2 with sync  pulsesel=Counter equals to zero (CTR=Zero)  blankinv=off  blankoffset=0  blankwidth=0  evsrcsel=Filtered version of DCAEVT1 (DCAEVT1FILT)  encape=off
  encoder_CH1 : c280xlib/eQEP  useModule=eQEP1  pcInputmode=Quadrature-count  externalClockrate=2x resolution: Count the rising/falling edge  swapPolarityselection=Clockwise  qdfOutputport=off  qapPolarityselection=off  qbpPolarityselection=off  qipPolarityselection=off  qspPolarityselection=off  igatePolarityselection=off  sampleTime=Tw  pcOutputport=on  pcMaximumvalue=4294967295  indexInitializationcheck=off  indexInitializationevent=Rising edge  strobeInitializationcheck=off  strobeInitializationevent=Rising edge  softwareInitializationcheck=on  softwareInitializationsource=Set to init value at start up  softwareInitializationmode=on  pcInitialvalue=0  pcResetmode=Reset on the maximum position  ieloutputport=off  indexEventlatch=Rising edge  seloutputport=off  strobeEventlatch=Rising edge  pcefOutputport=off  enableEqepcapture=off  qctmrOutputport=off  qcprdOutputport=off  captureTimerprescaler=1  upEventprescaler=1  overflowErrorflag=off  directionErrorflag=off  captureTimerposition=On unit time-out event  unitTimerperiod=100000000*0+4294967295  captureTimerlatch=off  capturePeriodlatch=off  positionCounterlatch=on  soenPolarityselection=off  spselPolarityselection=Index pin is used for sync output  compareValuesource=Specify via dialog  shadowMode=Load on QPOSCNT=0  compareValue=4294967295  syncOutputwidth=1  polaritySyncoutput=Active high  watchdogEnable=off  watchdogTimer=65535  outport1Datatype=auto  outport2Datatype=int32  outport3Datatype=auto  outport4Datatype=auto  outport5Datatype=auto  outport6Datatype=uint32  outport7Datatype=uint32  outport8Datatype=auto  outport9Datatype=auto  outport10Datatype=auto  outport11Datatype=auto  outport12Datatype=auto  eqepinterrupt_pce=off  eqepinterrupt_qpe=off  eqepinterrupt_qdc=off  eqepinterrupt_wto=off  eqepinterrupt_pcu=off  eqepinterrupt_pco=off  eqepinterrupt_pcr=off  eqepinterrupt_pcm=off  eqepinterrupt_sel=off  eqepinterrupt_iel=off  eqepinterrupt_uto=off  pheOutputport=off  watchdogOutputport=off  outport13Datatype=auto  outport14Datatype=auto
  potentiometer : c2802xlib/ADC  blkParamProc=C2000  ADCModule=1  samplingMode=Single sample mode  ADCResolution=12-bit (Single-ended input)  useSOC1=SOC4  useSOC2=SOC0_SOC1  SOCAcquisitionWindow=7  SOCTriggerSource=CPU0_TINT0n  SOCInterruptTrigger=No ADCINT  Ts=Ts*10  dType=single  postInterrupt=off  interruptSel=ADCINT1  ADCINTContinuous=on  endma=off  chdma=1  conv1=ADCINB7  conv2=ADCINA0 and ADCINB0  conv1_Type4=ADCIN0  conv2_Type4=ADCIN0 and ADCIN1
  Encoder [count] : Outport
  Encoder [count/s] : Outport  Port=2
  Rod angle [rad] : Outport  Port=3
  wires:
  Constant4/1 -> Add2/2
  Add3/1 -> Data Type Conversion12/1
  Data Type Conversion14/1 -> Add3/1, Scope5/1
  Saturation2/1 -> Data Type Conversion10/1
  Data Type Conversion13/1 -> Add2/1, Scope4/1
  Data Type Conversion10/1 -> ePWM4/1, Display5/1, ePWM3/1
  current sense A 8301 M2/1 -> Data Type Conversion14/1
  Data Type Conversion11/1 -> Gain10/1
  Data Type Conversion12/1 -> Gain11/1
  Gain10/1 -> Display6/1
  Gain11/1 -> Display7/1
  Delay/1 -> Subtract/2
  Add2/1 -> Data Type Conversion11/1
  Constant5/1 -> Add3/2
  current sense B 8301 M2/1 -> Data Type Conversion13/1
  Gain9/1 -> Saturation2/1
  encoder_CH1/1 -> Data Type Conversion1/1, Subtract/1, Delay/1
  Subtract/1 -> Data Type Conversion8/1
  "BLUE LED (0=off, 1=on)"/1 -> Digital Output1/1
  Constant7/1 -> Sum1/2
  Gain12/1 -> Sum1/1
  Sum1/1 -> Gain9/1
  Switch/1 -> Digital Output2/1
  ENABLE/1 -> Switch/2
  Constant8/1 -> Switch/1
  Constant9/1 -> Switch/3
  Saturation3/1 -> Gain12/1
  control [+/-1]/1 -> Saturation3/1
  Data Type Conversion8/1 -> Encoder [count/s]/1
  Data Type Conversion1/1 -> Encoder [count]/1
  potentiometer/1 -> Gain/1
  Gain/1 -> Rod angle [rad]/1

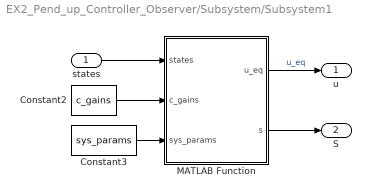
== system EX2_Pend_up_Controller_Observer/Subsystem/Subsystem1 ==
  states : Inport
  Constant2 : Constant  Value=c_gains
  Constant3 : Constant  Value=sys_params
  MATLAB Function : MATLAB Function  TreatAsAtomicUnit=on
  u : Outport
  S : Outport  Port=2
  wires:
  MATLAB Function/2(s) -> S/1
  states/1 -> MATLAB Function/1(states)
  Constant3/1 -> MATLAB Function/3(sys_params)
  Constant2/1 -> MATLAB Function/2(c_gains)
  MATLAB Function/1(u_eq) -> u/1  "u_eq"

== stateflow chart EX2_Pend_up_Controller_Observer/Safety StateFlow ==
  state RecoverFrom_UpperBound
    state Halt
      entry: u_out = 0;
    state HomingPulse
      entry:
      u_out = -0.2;
    state PostHomingWait
      entry:
      u_out = 0;
    state wait
      entry:
      flag = 1;
    (default) -> RecoverFrom_UpperBound.Halt
    RecoverFrom_UpperBound.Halt -> RecoverFrom_UpperBound.HomingPulse : [after(3,sec)]
    RecoverFrom_UpperBound.PostHomingWait -> RecoverFrom_UpperBound.wait : [after(3,sec)]
    RecoverFrom_UpperBound.HomingPulse -> RecoverFrom_UpperBound.PostHomingWait : [after(PULSE_TIME,sec)]
  state NormalOpertaion
    u_out = u_in;
    flag=0;
  state RecoverFrom_LowerBound
    state Halt
      entry: u_out = 0;
    state HomingPulse
      entry:
      u_out = 0.2;
    state PostHomingWait
      entry:
      u_out = 0;
    state wait
      entry:
      flag = 1;
    (default) -> RecoverFrom_LowerBound.Halt
    RecoverFrom_LowerBound.Halt -> RecoverFrom_LowerBound.HomingPulse : [[after(3,sec)]]
    RecoverFrom_LowerBound.HomingPulse -> RecoverFrom_LowerBound.PostHomingWait : [[after(PULSE_TIME,sec)]]
    RecoverFrom_LowerBound.PostHomingWait -> RecoverFrom_LowerBound.wait : [[after(3,sec)]]
  RecoverFrom_UpperBound -> NormalOpertaion : [flag==1]
  NormalOpertaion -> RecoverFrom_UpperBound [order 1] : [pos_s>0.25]
  (default) -> NormalOpertaion
  RecoverFrom_LowerBound -> NormalOpertaion : [[flag==1]]
  NormalOpertaion -> RecoverFrom_LowerBound [order 2] : [pos_s<-0.25]
  data: pos_s input; u_in input; PULSE_TIME constant double =1.8; u_out output; flag local =0

== matlab function EX2_Pend_up_Controller_Observer/Subsystem/Subsystem1/MATLAB Function ==
  data: states input; u_eq output; c_gains input; sys_params input; s output
function [u_eq, s] = calculate_u_eq(states, c_gains, sys_params)
% Calculates the equivalent control (u_eq) for a cart-pendulum system
% using the Sliding Mode Control formulation F_eq = -H/G.
% This function is derived from the full system equations provided.
%
% INPUTS:
%   states:     A vector of the system's current state [x, x_dot, theta, theta_dot]
%               Note: x is not used in this calculation, but is often part of the state vector.
%   c_gains:    A vector of the sliding surface gains [k1, k2, k3, k4] or [c1, c2, c3, c4]
%   sys_params: A vector of the system's physical parameters [M, m, L, I, b, g]
%
% OUTPUT:
%   u_eq:       The calculated equivalent control force.

% --- Unpack Inputs for Readability ---

% Unpack the state vector
x = states(1); % Not needed for this calculation
x_dot = states(2);
theta = states(3);
theta_dot = states(4);

% Unpack the sliding surface gains
k1 = c_gains(1); % Gain for position error (x - xd)
k2 = c_gains(2); % Gain for velocity error (x_dot)
k3 = c_gains(3); % Gain for angle error (theta)
k4 = c_gains(4); % Gain for angular velocity error (theta_dot)

% Unpack the system's physical parameters
M = sys_params(1); % Mass of the cart
m = sys_params(2); % Mass of the pendulum
L = sys_params(3); % Length of the pendulum
I = sys_params(4)+m*(L/2)^2; % Moment of inertia of the pendulum about its center
b = sys_params(5); % Friction coefficient for the cart
b_p = sys_params(6);
g = sys_params(7); % Acceleration due to gravity
K_sw = sys_params(8);
Kf_avg = 18.9500;
% --- Pre-calculate Common Terms for Efficiency ---
s_theta = sin(theta);
c_theta = cos(theta);
L_half = L / 2;

% Calculate the determinant of the mass matrix 'A' from our derivation
% det(A) = I(M + m) - (m^2 * L^2 / 4) * cos^2(theta)
detA = I * (M + m) - (m^2 * L^2 / 4) * c_theta^2;

% --- Decompose Dynamics into the form: ---
% x_ddot   = f1 + g1 * F
% theta_ddot = f2 + g2 * F

% For x_ddot:
term1_f1 = I * (m * L_half * theta_dot^2 * s_theta - b * x_dot);
term2_f1 = - (m * L_half * c_theta) * (m * g * L_half * s_theta - b_p * theta_dot);
f1 = (term1_f1 + term2_f1) / detA;
g1 = Kf_avg*I / detA;

% For theta_ddot:
term1_f2 = -(m * L_half * c_theta) * (m * L_half * theta_dot^2 * s_theta - b * x_dot);
term2_f2 = (M + m) * (m * g * L_half * s_theta - b_p * theta_dot);
f2 = (term1_f2 + term2_f2) / detA;
g2 = -Kf_avg*(m * L_half * c_theta) / detA;

% --- Calculate H and G from s_dot = H + G*F ---
% s_dot = k1*x_dot + k2*x_ddot + k3*theta_dot + k4*theta_ddot
% s_dot = k1*x_dot + k2*(f1 + g1*F) + k3*theta_dot + k4*(f2 + g2*F)
% s_dot = (k1*x_dot + k2*f1 + k3*theta_dot + k4*f2) + (k2*g1 + k4*g2)*F
% So, H = (numerator) and G = (denominator)

F = k1*x_dot + k2*f1 + k3*theta_dot + k4*f2;
G = k2*g1 + k4*g2;
s = k1*x + k2*x_dot + k3*theta + k4*theta_dot;
% h = -K_sw * sign(s);
h = -K_sw * tanh(100*s);
% --- Calculate u_eq = -H/G ---

% Avoid division by zero, which can happen if theta = +/- 90 degrees
% if the controller gains k2 and k4 are chosen poorly.
if abs(G) < 1e-9
    u_eq = 0; % Or a safe default value
else
    u_eq = (-F + h) / G;
end

end



% 
% 
% 
% function u_eq = calculate_u_eq(states, c_gains, sys_params)
% % Unpack inputs
% x_dot = states(2);
% theta = states(3);
% theta_dot = states(4);
% 
% c1 = c_gains(1);
% c2 = c_gains(2);
% c3 = c_gains(3);
% c4 = c_gains(4);
% 
% M = sys_params(1);
% m = sys_params(2);
% l = sys_params(3);
% g = sys_params(4);
% 
% % Pre-calculate common terms for efficiency
% s_theta = sin(theta);
% c_theta = cos(theta);
% D = M + m*s_theta^2;
% 
% % Calculate the dynamic terms from the EOMs
% f1 = (m*l*s_theta*theta_dot^2 - m*g*s_theta*c_theta) / D;
% g1 = 1 / D;
% 
% f2 = ((M+m)*g*s_theta - m*l*c_theta*s_theta*theta_dot^2) / (l*D);
% g2 = -c_theta / (l*D);
% 
% % Calculate u_eq based on setting sigma_dot = 0
% numerator = c2*f1 + c4*f2 + c1*x_dot + c3*theta_dot;
% denominator = c2*g1 + c4*g2;
% 
% % Avoid division by zero, although it's unlikely for this system
% if abs(denominator) < 1e-6
%     u_eq = 0;
% else
%     u_eq = -numerator / denominator;
% end
% 
% end

== stateflow chart EX2_Pend_up_Controller_Observer/Chart1 ==
  state Calibrating
    entry:
    u_out = 0;
    is_calibrated = 0;
  state Controlling
    entry:
    is_calibrated = 1;
    during:
    u_out = u_from_ctrl;
  (default) -> Calibrating
  Calibrating -> Controlling : after(CALIBRATION_TIME, sec)
  data: u_from_ctrl input; u_out output; is_calibrated output; CALIBRATION_TIME constant double =50
